simulink model "acc_RR_backup"  (R2021b)
settings: Solver=FixedStepAuto  StartTime=0.0  StopTime=40  FixedStep=0.0005  RelTol=1e-3
values from neighbouring files (symbols this model uses):
  s_path = [0 1.10508939428 2.2141958029 3.32141571172 4.42705301151 5.53154548532 6.63517443471 7.73808041313 8.84055018688 9.94289959674 11.0453539299 12.1480581097 ... (1001 elements, 1001x1)]    [200_100radius.mat]    (also in LV_Clothoid_S_Turn_path.mat = [0 0.966832089581 1.93621320584 2.90214024471 3.86476766313 ; NEDC_path.mat = [0 0.414605943146 0.832514087334 1.25401518562 1.68216660344; Straight_East_into_curve.mat = [0 1.65770560069 3.32192925577 4.98420060507 6.64484613518 8; acc_plot_backup.m = Station_HV_m)
  X_path = [0 1.10508939428 2.2141958029 3.32141571172 4.42705301151 5.53154548532 6.63517443471 7.73808041313 8.84055018688 9.94289959674 11.0453539299 12.1480581097 ... (1001 elements, 1001x1)]    [200_100radius.mat]    (also in LV_Clothoid_S_Turn_path.mat = [-10 -9.03316791042 -8.06378679416 -7.09785975529 -6.1352323; NEDC_path.mat = [0 0.414605943146 0.832514087334 1.25401518562 1.68216660344; Straight_East_into_curve.mat = [0 1.65770560069 3.32192925577 4.98420060507 6.64484613518 8; acc_plot_backup.m = X_HV_m)
  Y_path = [0 -1.70364610795e-18 -7.41532896709e-18 1.46822109542e-17 4.74557362791e-17 6.12980216762e-17 9.25043977736e-17 1.24088240159e-16 1.5099156923e-16 1.7058517853e-16 1.90629227614e-16 2.09673434424e-16 ... (1001 elements, 1001x1)]    [200_100radius.mat]    (also in LV_Clothoid_S_Turn_path.mat = [0 -8.46153035536e-19 5.07382551045e-18 2.07356032218e-17 3.; NEDC_path.mat = [0 -3.50680326162e-18 -2.14111304971e-18 3.38197671014e-18 3; Straight_East_into_curve.mat = [0 1.29197709199e-18 2.81882429322e-18 3.49020462564e-17 6.7; acc_plot_backup.m = Y_HV_m)
undefined symbols (not defined in the file or in its folder): C_TICK_TIME_S, ENUM_ACCSTATE_DISABLED, ENUM_ACCSTATE_OFF, ENUM_ACCSTATE_STANDBY, FALSE, KVDI_ACCLongPressTime_ms, KVDI_ACCMaxActSpeed_kph, KVDI_ACCSetSpdIntial_kph, KVDI_ACCSpdLargeChange_kph, KVDI_LongPressConTime_ms, ONE_FLOAT, ONE_INT, R, Rw, T, TRUE, ZERO_FLOAT, ZERO_INT
libraries: simulink x15, simulink_extras x2, Solver_SF x1
(part 1 of 4)
settings Model: Creator=power  LastModifiedBy=power
settings DataIOCC: ReturnWorkspaceOutputs=off

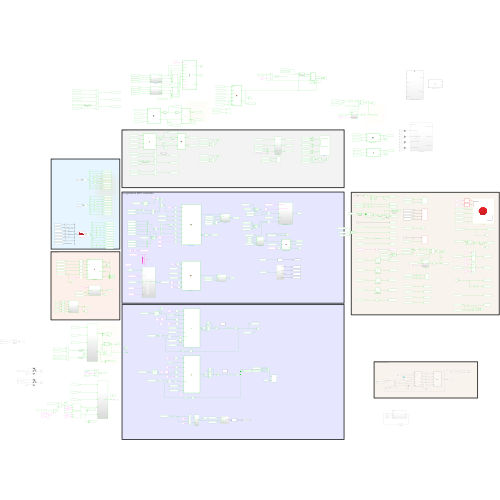
[thumbnail: Simulink's stored preview of the top-level diagram]
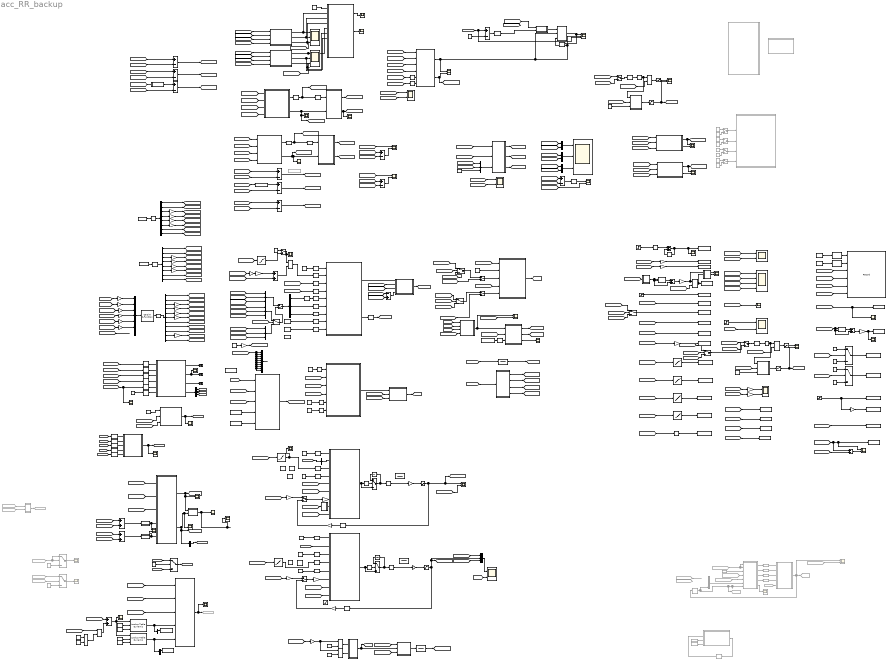
== system acc_RR_backup ==
  note: Lateral MPC controller
  note: Kalman Filter
  note: Carsim
  note: Record data
  note: Longitudinal MPC controller
  note: Camera_emulator
  note: Longitudinal Constraint MPC controller
  1-D Lookup Table : Lookup_n-D  NumberOfTableDimensions=1  BreakpointsForDimension1=[-10:1]  Table=[2.4 2.4 2.3 2.2 2.1 2.0 1.9 1.8 1.7 1.6 1.5 1.5]  InternalRulePriority=Speed  RndMeth=Simplest  InputSameDT=on
  1-D Lookup Table Accel Limit1 : Lookup_n-D  NumberOfTableDimensions=1  BreakpointsForDimension1=[0,5,20,30]  Table=[4,4,2,2]  InternalRulePriority=Speed  RndMeth=Simplest  InputSameDT=on
  1-D Lookup Table Deccel Limit2 : Lookup_n-D  NumberOfTableDimensions=1  BreakpointsForDimension1=[0,5,20,30]  Table=[-5,-5,-2.5,-2.5]  InternalRulePriority=Speed  RndMeth=Simplest  InputSameDT=on
  1-D Lookup Table Jerk LowLimit1 : Lookup_n-D  NumberOfTableDimensions=1  BreakpointsForDimension1=[0,5,20,30]  Table=[-5,-5,-2.5,-2.5]  InternalRulePriority=Speed  RndMeth=Simplest  InputSameDT=on
  1-D Lookup Table Jerk UpLimit1 : Lookup_n-D  NumberOfTableDimensions=1  BreakpointsForDimension1=[0,5,20,30]  Table=[5,5,2.5,2.5]  InternalRulePriority=Speed  RndMeth=Simplest  InputSameDT=on
  1-D Lookup Table1 : Lookup_n-D  NumberOfTableDimensions=1  BreakpointsForDimension1=[35 40 70 80]/3.6  Table=[0.01 0.01 0.0025 0.0025]  InternalRulePriority=Speed  RndMeth=Simplest  InputSameDT=on
  1-D Lookup Table2 : Lookup_n-D  NumberOfTableDimensions=1  BreakpointsForDimension1=[0 10 35 40]/3.6  Table=[0.25 0.25 0.025 0.025]  InternalRulePriority=Speed  RndMeth=Simplest  InputSameDT=on
  ACCSpdCalculation : Subsystem  Commented=on
  ACC_Mode_Selector : Subsystem
  Abs{,1..3} (4 alike) : Abs
  Acceleration controller2 : MATLAB Function  TreatAsAtomicUnit=on
  Add{,1..3,5,13..18} (11 alike) : Sum  Inputs=+-
  Add Constant : Bias  Bias=-2
  Add Constant1 : Bias  Bias=2
  Add Constant2 : Bias  Bias=-2
  Add Constant3 : Bias  Bias=-4.5
  Add10 : Sum  Inputs=-+
  Add{6..9,11} (5 alike) : Sum
  Add12 : Sum  Inputs=-+
  Add4 : Sum  Inputs=-+
  Camera_NEW : MATLAB Function  TreatAsAtomicUnit=on
  CarSim S-Function : Solver_SF/CarSim S-Function  Priority=1  SIMFILE=simfile.sim  Run_RTs=off  vs_state_ind=Run  StopMode_ind=Vehicle Model
  Compare To Constant : simulink/Logic and Bit Operations/Compare To Constant  relop=<=  const=-0.2  OutDataTypeStr=boolean
  Constant{,8..9,16,19,28,40,42,52,58,92} (11 alike) : Constant
  Constant1 : Constant  Value=0
  Constant10 : Constant  Value=0.1
  Constant11 : Constant  Value=90
  Constant111 : Constant  Value=10
  Constant{12..13,24,45} (4 alike) : Constant  Commented=on  OutDataTypeStr=boolean
  Constant14 : Constant  Value=1270+22*4+88.6+54.4
  Constant{15,39,46..47} (4 alike) : Constant  Commented=on  Value=0  OutDataTypeStr=boolean
  Constant17 : Constant  Value=0.3
  Constant18 : Constant  Value=0.025
  Constant2 : Constant  Value=2
  Constant20 : Constant  Value=s_path
  Constant21 : Constant  Value=X_path
  Constant22 : Constant  Value=s_path
  Constant23 : Constant  Value=Y_path
  Constant25 : Constant  Commented=on  Value=0.3
  Constant26 : Constant  Value=X_path
  Constant27 : Constant  Value=Y_path
  Constant29 : Constant  Value=1.5
  Constant3 : Constant  Value=0.1
  Constant30 : Constant  Value=35
  Constant31 : Constant  Value=3
  Constant32 : Constant  Value=30
  Constant33 : Constant  Value=5
  Constant34 : Constant  Value=-3
  Constant35 : Constant  Value=-5
  Constant36 : Constant  Value=1.5
  Constant37 : Constant  Commented=on  Value=0.1
  Constant38 : Constant  Value=0.025
  Constant4 : Constant  Value=0.0025
  Constant41 : Constant  Value=0.01
  Constant43 : Constant  Value=0.0125
  Constant44 : Constant  Commented=on  Value=100
  Constant48 : Constant  Commented=on  Value=100
  Constant49 : Constant  Value=[1:10]'
  Constant5 : Constant  Value=0.2
  Constant50 : Constant  Commented=on  Value=3
  Constant51 : Constant  Value=0.1
  Constant53 : Constant  Value=1.5
  Constant6 : Constant  Value=2.5
  Constant7 : Constant  Value=0
  Delay{,3..4,7} (4 alike) : Delay  DelayLength=1  SampleTime=0.1
  Delay1 : Delay  DelayLength=1  InitialConditionSource=Input port  SampleTime=0.1
      settings: InputPortMap=u0,p4
  Delay2 : Delay  DelayLength=1  InitialConditionSource=Input port  SampleTime=0.1
      settings: InputPortMap=u0,p4
  Delay5 : Delay  Commented=on  DelayLength=1  SampleTime=0.1
  Delay6 : Delay  DelayLength=1  InitialConditionSource=Input port  SampleTime=0.1
      settings: InputPortMap=u0,p4
  Delay8 : Delay  Commented=on  DelayLength=1  SampleTime=0.1
  Demux : Demux  Outputs=11
  Demux1 : Demux  Outputs=8
  Demux14 : Demux
  Demux2 : Demux  Outputs=[10]
  Demux3 : Demux  Outputs=3
  Demux4 : Demux  Outputs=[1 9]
  Demux5 : Demux  Outputs=[1 9]
  Demux6 : Demux  Outputs=[8 10 12]
  Demux7 : Demux  Outputs=8
  Divide : Product  Inputs=*/
  Divide1 : Product  Inputs=*/
  Estimation_TTCx_PV : MATLAB Function  TreatAsAtomicUnit=on
  Estimation_TTCx_PV1 : MATLAB Function  TreatAsAtomicUnit=on
  Estimation_TTCy_PV : MATLAB Function  Commented=on  TreatAsAtomicUnit=on
  From Workspace : FromWorkspace  VariableName=LV
  From Workspace1 : FromWorkspace  VariableName=APV
  From149 : From  Commented=on  GotoTag=Ax_HV_mps2
  From157 : From  Commented=on  GotoTag=Vx_p
  From159 : From  Commented=on  GotoTag=ACCSetSpeed_mps
  From160 : From  Commented=on  GotoTag=Vx_HV_mps
  From161 : From  Commented=on  GotoTag=Ax_HV_mps2
  From163 : From  Commented=on  GotoTag=RR
  From165 : From  Commented=on  GotoTag=xref
  From166 : From  Commented=on  GotoTag=yref
  From167 : From  Commented=on  GotoTag=xref
  From169 : From  Commented=on  GotoTag=xref
  From170 : From  Commented=on  GotoTag=yref
  From245 : From  Commented=on  GotoTag=ax_c_old
  Gain{1..2,5,9..10,15..16} (7 alike) : Gain  Gain=1/3.6
  Gain{3..4,6..7,11,29} (6 alike) : Gain  Gain=9.81
  Gain12 : Gain  Gain=0.5
  Gain{8,13,19..21,31} (6 alike) : Gain  Gain=3.6
  Gain14 : Gain  Gain=pi/180
  Gain17 : Gain  Gain=0.1
  Gain18 : Gain  Gain=[0:9]
  Gain22 : Gain  Gain=0.5
  Gain23 : Gain  Gain=20
  Gain{24..26,34} (4 alike) : Gain  Gain=1/20
  Gain27 : Gain  Gain=pi/180
  Gain28 : Gain  Gain=20
  Gain30 : Gain  Gain=pi/180
  Gain{33,36..38} (4 alike) : Gain
  Gain35 : Gain  Gain=-1
  Goto31 : Goto  Commented=on  GotoTag=ax_c_old
  Goto44 : Goto  Commented=on  GotoTag=spd_acc
  Goto46 : Goto  Commented=on  GotoTag=LeftDis_Camera
  Goto49 : Goto  Commented=on  GotoTag=LeftDis_PV
  Latch : Subsystem
  Logical Operator : Logic  Operator=NOT  AllPortsSameDT=off  OutDataTypeStr=boolean
  Lookup Table Dynamic : simulink/Lookup Tables/Lookup Table Dynamic  LookUpMeth=Interpolation-Use End Values  OutDataType=fixdt('double')  OutScaling=[]  OutputDataTypeScalingMode=Specify via dialog  OutDataTypeStr=double  DoSatur=off
  Lookup Table Dynamic1 : simulink/Lookup Tables/Lookup Table Dynamic  LookUpMeth=Interpolation-Use End Values  OutDataType=fixdt('double')  OutScaling=[]  OutputDataTypeScalingMode=Specify via dialog  OutDataTypeStr=double  DoSatur=off
  MATLAB Function : MATLAB Function  TreatAsAtomicUnit=on
  MATLAB Function1 : MATLAB Function  TreatAsAtomicUnit=on
  MATLAB Function10 : MATLAB Function  TreatAsAtomicUnit=on
  MATLAB Function13 : MATLAB Function  TreatAsAtomicUnit=on
  MATLAB Function17 : MATLAB Function  TreatAsAtomicUnit=on
  MATLAB Function2 : MATLAB Function  TreatAsAtomicUnit=on
  MATLAB Function3 : MATLAB Function  TreatAsAtomicUnit=on
  MATLAB Function4 : MATLAB Function  TreatAsAtomicUnit=on
  MATLAB Function5 : MATLAB Function  TreatAsAtomicUnit=on
  MATLAB Function6 : MATLAB Function  TreatAsAtomicUnit=on
  MATLAB Function7 : MATLAB Function  TreatAsAtomicUnit=on
  MATLAB Function8 : MATLAB Function  TreatAsAtomicUnit=on
  MPC : MATLAB Function  Commented=on  TreatAsAtomicUnit=on
  MPC_ACC : MATLAB Function  TreatAsAtomicUnit=on
  MPC_Bicycle_LDC1 : MATLAB Function  TreatAsAtomicUnit=on
  Manual Switch : ManualSwitch  Commented=on
  Manual Switch1 : ManualSwitch  CurrentSetting=0
  Manual Switch10 : ManualSwitch  Commented=on  CurrentSetting=0
  Manual Switch11 : ManualSwitch  Commented=on
  Manual Switch12 : ManualSwitch  Commented=on
  Manual Switch{2..6,8..9} (7 alike) : ManualSwitch
  Mux : Mux  Inputs=7
  Mux1 : Mux  Inputs=2
  Mux{4,6..8,10} (5 alike) : Mux  Inputs=3
  Mux2 : Mux  Inputs=2
  Mux3 : Mux  Inputs=2
  Mux5 : Mux  Inputs=10
  Mux9 : Mux  Commented=on  Inputs=[3 1 1 1]
  Product : Product
  Product1 : Product
  Product10 : Product
  QP_logitudinal1 : MATLAB Function  Commented=on  TreatAsAtomicUnit=on
  R1 : Constant  Value=0.5
  Radians to Degrees1 : simulink_extras/Transformations/Radians to Degrees
  Radians to Degrees2 : simulink_extras/Transformations/Radians to Degrees
  Rate Transition{1..5,18} (6 alike) : RateTransition  OutPortSampleTime=0.1
  Relational Operator : RelationalOperator  OutDataTypeStr=boolean  RndMeth=Simplest
  Relational Operator1 : RelationalOperator  Operator=<=  OutDataTypeStr=boolean  RndMeth=Simplest
  Relational Operator2 : RelationalOperator  Operator=isNaN  OutDataTypeStr=boolean  RndMeth=Simplest
  Relational Operator4 : RelationalOperator  Operator=isNaN  OutDataTypeStr=boolean  RndMeth=Simplest
  Saturation{,1,5..6} (4 alike) : Saturate  UpperLimit=2.5  LowerLimit=0
  Saturation2 : Saturate  UpperLimit=30/3.6  LowerLimit=5/3.6
  Saturation3 : Saturate  UpperLimit=720  LowerLimit=-720
  Saturation4 : Saturate  UpperLimit=400  LowerLimit=-400
  Scope{,1..2,5,8,13,17..20,25,27..28,30,42..44,46,67} (19 alike) : Scope  NumInputPorts=2
  Scope{3..4,6..7,9..10,14..16,22..24,26,29,31..32,35,37,39,41,45,159} (22 alike) : Scope
  Scope{11,36,40,47} (4 alike) : Scope  NumInputPorts=3
  Scope12 : Scope  NumInputPorts=4
  Scope21 : Scope  Commented=on  NumInputPorts=2
  Scope33 : Scope  Commented=on
  Scope34 : Scope  Commented=on
  Scope38 : Scope  Commented=on
  Smooth Switch : Subsystem
  Smooth Switch1 : Subsystem
  Step : Step  Time=0  Before=1.5  After=1.5  SampleTime=0
  Step1 : Step  Time=0  Before=1.5  After=1.5  SampleTime=0
  Step2 : Step  Time=0  After=0.1  SampleTime=0
  Step3 : Step  Time=0  Before=5  After=5  SampleTime=0.1
  Subsystem : Subsystem
  Subsystem1 : Subsystem
  Subsystem16 : Subsystem
  Subsystem17 : Subsystem
  Subsystem2 : Subsystem
  Subsystem20 : Subsystem
  Subsystem3 : Subsystem
  Subsystem4 : Subsystem
  Subsystem5 : Subsystem
  Subsystem6 : Subsystem  Commented=on
  Subsystem7 : Subsystem
  Subsystem8 : Subsystem
  Switch : Switch  Criteria=u2 > Threshold
  Switch{1,7..11} (6 alike) : Switch  Criteria=u2 ~= 0
  Switch2 : Switch  Commented=on  Criteria=u2 > Threshold
  Switch3 : Switch  Commented=on  Criteria=u2 > Threshold
  Switch4 : Switch  Criteria=u2 > Threshold
  Switch5 : Switch  Threshold=8
  Switch6 : Switch  Threshold=8
  TH_ref : Constant  Value=1.5
  Terminator1 : Terminator
  Terminator2 : Terminator
  Terminator3 : Terminator
  To Workspace : ToWorkspace  VariableName=X_HV_m  SampleTime=-1
  To Workspace1 : ToWorkspace  VariableName=Y_HV_m  SampleTime=-1
  To Workspace10 : ToWorkspace  VariableName=TH  SampleTime=-1
  To Workspace11 : ToWorkspace  VariableName=RR  SampleTime=-1
  To Workspace12 : ToWorkspace  VariableName=Desired_distance  SampleTime=-1
  To Workspace13 : ToWorkspace  VariableName=C_tick_time  SampleTime=-1
  To Workspace14 : ToWorkspace  VariableName=Ax_HV_mps2  SampleTime=-1
  To Workspace15 : ToWorkspace  VariableName=V_ref_kph  SampleTime=-1
  To Workspace16 : ToWorkspace  VariableName=Ax_Up_Limit  SampleTime=-1
  To Workspace17 : ToWorkspace  VariableName=Ax_Low_Limit  SampleTime=-1
  To Workspace18 : ToWorkspace  VariableName=Jerk_x_Up_Limit  SampleTime=-1
  To Workspace19 : ToWorkspace  VariableName=Jerk_x_Low_Limit  SampleTime=-1
  To Workspace2 : ToWorkspace  VariableName=Yaw_HV_deg  SampleTime=-1
  To Workspace20 : ToWorkspace  VariableName=Acc_Mode  SampleTime=-1
  To Workspace21 : ToWorkspace  VariableName=Ay_Low_Limit  SampleTime=-1
  To Workspace22 : ToWorkspace  VariableName=Jerk_y_Up_Limit  SampleTime=-1
  To Workspace23 : ToWorkspace  VariableName=Jerk_y_Low_Limit  SampleTime=-1
  To Workspace24 : ToWorkspace  VariableName=Ay_HV_mps2  SampleTime=-1
  To Workspace25 : ToWorkspace  VariableName=y_error  SampleTime=-1
  To Workspace26 : ToWorkspace  VariableName=Steer_SW_deg  SampleTime=-1
  To Workspace27 : ToWorkspace  VariableName=X_ref  SampleTime=-1
  To Workspace28 : ToWorkspace  VariableName=Y_ref  SampleTime=-1
  To Workspace3 : ToWorkspace  VariableName=Station_HV_m  SampleTime=-1
  To Workspace4 : ToWorkspace  VariableName=Jerk_y  SampleTime=-1
  To Workspace5 : ToWorkspace  VariableName=Ay_Up_Limit  SampleTime=-1
  To Workspace6 : ToWorkspace  VariableName=HV_kph  SampleTime=-1
  To Workspace7 : ToWorkspace  VariableName=PV_kph  SampleTime=-1
  To Workspace8 : ToWorkspace  VariableName=Jerk_x  SampleTime=-1
  To Workspace9 : ToWorkspace  VariableName=TH_ref  SampleTime=0.1
  Transfer Fcn{1..4} (4 alike) : TransferFcn  Denominator=[0.3 1]
  Unit Delay : UnitDelay  SampleTime=-1  HasFrameUpgradeWarning=on
  Unit Delay2 : UnitDelay  SampleTime=-1  HasFrameUpgradeWarning=on
  V_rel Estimation : Subsystem
  XY Graph : Record  FileSettingsInternal="{\"entries\":[{\"content\":{\"excelSettings\":{\"content\":{},\"type\":\"Streamout.ExcelSettings\"}},\"type\":\"Streamout.FileSettingStorage\",\"uuid\":\"a3c8dcb7-cd04-47db-8df7-74fc07aaeb0b\"}],\"packageUris\":[\"http://schema.mathworks.com/mf0/streamout_blocks/R2020a\"],\"version\":\"1.0\"}"  Layout=[1 1]  SignalsInternal="{\"entries\":[{\"content\":{\"signals\":[{\"content\":{\"blockPath\":[\"acc/XY Graph\"],\"channel\":[],\"dimensions\":[1],\"domain\":\"acc/XY Graph\",\"lineColor\":\"#a2142f\",\"plots\":[1],\"port\":1,\"sid\":[\"\"],\"signalID\":328902,\"signalName\":\"x\"},\"type\":\"RecordBlkView.Signal\",\"uuid\":\"58a908f8-b328-4002-bf13-044fef450135\"},{\"content\":{\"blockPath\":[\"acc/XY Graph\"],\"channel\":[],\"dimensions\":[1],\"domain\":\"acc/XY Graph\",\"lineColor\":\"#139fff\",\"plots\":[1],\"port\":2,\"sid\":[\"\"],\"signalID\":328906,\"signalName\":\"y\"},\"type\":\"RecordBlkView.Signal\",\"uuid\":\"8476c32c-9a1a-438a-a83a-d74f9b55deb6\"},{\"content\":{\"blockPath\":[\"acc/XY Graph\"],\"channel\":[],\"dimensions\":[1],\"domain\":\"acc/XY Graph\",\"lineColor\":\"#64d413\",\"plots\":[1],\"port\":3,\"sid\":[\"\"],\"signalID\":328910,\"signalName\":\"X_HV\"},\"type\":\"RecordBlkView.Signal\",\"uuid\":\"60bc389a-c242-4b2e-b286-84b9602f93c9\"},{\"content\":{\"blockPath\":[\"acc/XY Graph\"],\"channel\":[],\"dimensions\":[1],\"domain\":\"acc/XY Graph\",\"lineColor\":\"#ff13a6\",\"plots\":[1],\"port\":4,\"sid\":[\"\"],\"signalID\":328914,\"signalName\":\"Y_HV\"},\"type\":\"RecordBlkView.Signal\",\"uuid\":\"a6cb8bdb-3617-4429-b963-4035cabf589a\"},{\"content\":{\"blockPath\":[\"acc/XY Graph\"],\"channel\":[],\"dimensions\":[1],\"domain\":\"acc/XY Graph\",\"lineColor\":\"#ff6929\",\"plots\":[1],\"port\":5,\"sid\":[\"\"],\"signalID\":328918,\"signalName\":\"X_PV\"},\"type\":\"RecordBlkView.Signal\",\"uuid\":\"139bb408-47f9-477b-b130-41a093de5c1a\"},{\"content\":{\"blockPath\":[\"acc/XY Graph\"],\"channel\":[],\"dimensions\":[1],\"domain\":\"acc/XY Graph\",\"lineColor\":\"#b746ff\",\"plots\":[1],\"port\":6,\"sid\":[\"\"],\"signalID\":328922,\"signalName\":\"Y_PV\"},\"type\":\"RecordBlkView.Signal\",\"uuid\":\"dcabd0e2-8491-473f-998f-2ebadf0b1da2\"}]},\"type\":\"RecordBlkView.InputSignals\",\"uuid\":\"b146c4fa-b7cd-488d-8ce9-66e4c4b64d1a\"}],\"packageUris\":[\"http://schema.mathworks.com/mf0/streamout_blocks/R2020a\"],\"version\":\"1.0\"}"  VisualizationBindings="{\"xyplotplugin\":{\"info\":[{\"series\":[{\"bindingParametersList\":[{\"parameter\":\"X-Axis\",\"signalID\":328902,\"signalName\":\"x\"},{\"parameter\":\"Y-Axis\",\"signalID\":328906,\"signalName\":\"y\"}],\"seriesID\":43394},{\"bindingParametersList\":[{\"parameter\":\"X-Axis\",\"signalID\":328918,\"signalName\":\"X_PV\"},{\"parameter\":\"Y-Axis\",\"signalID\":328922,\"signalName\":\"Y_PV\"}],\"seriesID\":18431},{\"bindingParametersList\":[{\"parameter\":\"X-Axis\",\"signalID\":328910,\"signalName\":\"X_HV\"},{\"parameter\":\"Y-Axis\",\"signalID\":328914,\"signalName\":\"Y_HV\"}],\"seriesID\":48931}],\"subplotID\":1}]}}"  CompatibilityTag=XY
  Zero-Order Hold{1..14,17..25,132..136} (28 alike) : ZeroOrderHold  SampleTime=0.1
  Zero-Order Hold{26..27,29,36} (4 alike) : ZeroOrderHold  Commented=on  SampleTime=0.1
  acceleration_apr1 : Subsystem
  acceleration_apr4 : Subsystem
  car_length : Bias  Bias=-4.5
  car_length1 : Bias  Bias=4.5
  car_length2 : Bias  Bias=-4.5
  car_length3 : Bias  Bias=4.5
  cmd_limiter2 : Subsystem
  cmd_limiter3 : Subsystem
  demux : Subsystem
  demux2 : Subsystem
  dist_safe : Bias  Bias=-2
  divide : Subsystem
  divide1 : Subsystem
  global to local1 : Subsystem
  global to local3 : Subsystem
  relative_dynamic_estimated : Subsystem  Commented=on
  rolling_avg : Subsystem  Commented=on
  sample time1 : Gain  Gain=1/0.1
  sample time2 : Gain  Gain=1/0.1
  velocity_apr5 : Subsystem  Commented=on
  wires:
  V_rel Estimation/3(a_rel) -> [a_Rel_est]
  [RR] -> V_rel Estimation/2(S_rel)
  [Ax_HV_mps2] -> V_rel Estimation/1(a_c)
  V_rel Estimation/1(s_rel) -> [S_Rel_est]
  Demux/1 -> [X_HV_m]
  CarSim S-Function/1 -> Zero-Order Hold18/1
  Demux/2 -> [Y_HV_m]
  Demux/3 -> Gain9/1
  Demux/4 -> Gain10/1
  Demux/5 -> Gain3/1
  Demux/6 -> Gain4/1
  From Workspace/1 -> Zero-Order Hold5/1
  Demux1/1 -> [X_PV_m]
  Demux1/6 -> Gain11/1
  Demux1/5 -> Gain7/1
  Demux1/4 -> Gain2/1
  Demux1/3 -> Gain1/1
  Demux1/2 -> [Y_PV_m]
  Divide/1 -> Saturation/1  "TH_cal"
  Saturation/1 -> Scope5/1  "TH"
  [Vx_PV_mps] -> Add1/1
  [Vx_HV_mps] -> Add1/2
  acceleration_apr4/1(acc_a) -> Add2/1  "PV"
  [Ax_HV_mps2] -> Add2/2  "HV"
  Constant14/1 -> Zero-Order Hold17/1
  Subsystem2/4(Pb_RR) -> [Braking_Pressure_RR]
  Product/1 -> Zero-Order Hold6/1
  [Driving_Brk_Cmd] -> Subsystem2/1(T_cmd)
  Subsystem2/1(Pb_LF) -> [Braking_Pressure_LF]
  Acceleration controller2/2(Tb) -> [Driving_Brk_Cmd]
  Acceleration controller2/3(Rtotal) -> Scope159/1
  Subsystem2/3(Pb_RL) -> [Braking_Pressure_RL]
  [Ax_HV_mps2] -> Zero-Order Hold9/1
  [Vx_HV_mps] -> Zero-Order Hold8/1
  Acceleration controller2/1(Tr) -> [Driving_Torque_Cmd]  "Torque"
  Subsystem2/2(Pb_RF) -> [Braking_Pressure_RF]
  Gain9/1 -> [Vx_HV_mps]
  Gain10/1 -> [Vy_HV_mps]
  Gain2/1 -> [Vy_PV_mps]
  Gain3/1 -> [Ax_HV_mps2]
  Gain4/1 -> [Ay_HV_mps2]
  Gain11/1 -> [Ay_PV_mps2]
  Gain22/1 -> Mux/1  "Driving_Torque_FL"
  Gain12/1 -> Mux/2  "Driving_Torque_FR"
  Zero-Order Hold6/1 -> MATLAB Function1/2(Yref)
  Zero-Order Hold8/1 -> MATLAB Function1/3(Vx)
  Zero-Order Hold9/1 -> MATLAB Function1/4(ax)
  Zero-Order Hold10/1 -> MATLAB Function1/5(D_rel)
  Zero-Order Hold11/1 -> MATLAB Function1/6(V_rel)
  Zero-Order Hold12/1 -> MATLAB Function1/7(ax_rel)
  Zero-Order Hold13/1 -> MATLAB Function1/8(Qs)
  Zero-Order Hold14/1 -> MATLAB Function1/9(Rs)
  Abs/1 -> divide/1(dividend), Divide/1
  Mux1/1 -> Scope11/1  "RR"
  [RR] -> Mux1/1  "RR"
  [S_Rel_est] -> Mux1/2  "Est"
  [RVx] -> Mux2/1  "RV"
  [V_Rel_est] -> Mux2/2  "Est"
  [RAx] -> Mux3/1  "RA"
  [a_Rel_est] -> Mux3/2  "Est"
  Mux2/1 -> Scope11/2  "RV"
  Mux3/1 -> Scope11/3  "RA"
  [Braking_Pressure_RF] -> Gain36/1
  Gain33/1 -> Mux/3  "Driving_Torque_LF"
  [Braking_Pressure_LF] -> Gain33/1
  [Braking_Pressure_RL] -> Gain37/1
  Gain36/1 -> Mux/4  "Driving_Torque_RF"
  Gain38/1 -> Mux/6  "Driving_Torque_RR"
  Gain37/1 -> Mux/5  "Driving_Torque_RL"
  [Braking_Pressure_RR] -> Gain38/1
  [Braking_Pressure_LF] -> Scope12/1  "LF"
  [Braking_Pressure_RF] -> Scope12/2  "RF"
  [Braking_Pressure_RL] -> Scope12/3  "RL"
  [Braking_Pressure_RR] -> Scope12/4  "RR"
  MATLAB Function1/2(Y) -> Add Constant1/1  "MPC"
  Gain8/1 -> Scope18/1  "HV"
  Gain13/1 -> Scope18/2  "PV"
  Zero-Order Hold5/1 -> Demux1/1
  [Vx_HV_mps] -> Acceleration controller2/2(Vxh)
  Zero-Order Hold17/1 -> Acceleration controller2/3(m)
  Zero-Order Hold18/1 -> Demux/1
  [RR] -> Scope13/2  "RR"
  [Vx_HV_mps] -> Divide/2
  Mux4/1 -> V_rel Estimation/3(initial_value)
  [RR] -> Mux4/1
  Constant7/1 -> Mux4/3
  Step/1 -> Scope2/1  "TH_limit"
  [TH] -> Scope2/2  "TH"
  Gain7/1 -> [Ax_PV_mps2]
  Demux3/3 -> Zero-Order Hold12/1
  Zero-Order Hold3/1 -> MATLAB Function1/1(mode)
  [Driving_Torque] -> Gain22/1
  [Driving_Torque] -> Gain12/1
  [Ax_HV_mps2] -> Scope17/2  "ax_out"
  [Vx_HV_mps] -> Gain8/1  "HV"
  [Vx_PV_mps] -> Gain13/1  "PV"
  Demux3/2 -> Zero-Order Hold11/1
  [Driving_Torque_Cmd] -> Transfer Fcn1/1
  Gain1/1 -> [Vx_PV_mps]
  [Vx_HV_mps] -> MPC_ACC/3(Vx)
  [Ax_HV_mps2] -> MPC_ACC/4(ax)
  Constant92/1 -> Zero-Order Hold1/1
  Constant5/1 -> Zero-Order Hold2/1
  Constant2/1 -> Subsystem/4(Ax_max)
  Constant6/1 -> Subsystem/5(Jx_max)
  [Vx_HV_mps] -> Subsystem/3(VehSpd)
  [Vx_p] -> MPC_ACC/2(vx_p)
  Subsystem/1("VREF_LongiVehSpdRef_mps ") -> [Vx_p]  "mps"
  Zero-Order Hold1/1 -> MPC_ACC/5(Qs)
  Zero-Order Hold2/1 -> MPC_ACC/6(Rs)
  V_rel Estimation/2(v_rel) -> [V_Rel_est]
  MATLAB Function1/1(u) -> cmd_limiter2/1(ax_cmd)  "cmd"
  [RVx] -> Mux4/2
  Constant28/1 -> Zero-Order Hold4/1
  Add2/1 -> [RAx]
  Add1/1 -> [RVx]
  [Acc_Mode] -> Subsystem/1("Trig ")
  [RR] -> ?
  [ACCSetSpeed_mps] -> Mux5/10, Mux5/9, Mux5/8, Mux5/7, Mux5/6, Mux5/5, Mux5/4, Mux5/3, Mux5/2, Mux5/1
  Add Constant/1 -> Abs/1
  Constant11/1 -> Gain15/1
  Gain15/1 -> [ACCSetSpeed_mps]
  Constant58/1 -> Zero-Order Hold3/1
  Demux3/1 -> dist_safe/1
  [ACCSetSpeed_mps] -> ACC_Mode_Selector/1(ACCSetSpeed_mps)
  Constant1/1 -> ACC_Mode_Selector/2(VACCTargetVehNotAssigned_flg)
  [RR] -> Switch9/3
  [Vx_HV_mps] -> ACC_Mode_Selector/4(Vx_HV_mps)
  [RVx] -> Switch8/3
  [Vx_HV_mps] -> Add6/2
  [Ax_HV_mps2] -> Gain17/1
  Gain17/1 -> Gain18/1
  Gain18/1 -> Add6/1
  Add6/1 -> Product/2  "Vp"
  Add Constant1/1 -> [Desired_distance]
  [Ax_PV_mps2] -> acceleration_apr4/1(acc_b)  "PV"
  Transfer Fcn1/1 -> [Driving_Torque]
  [Vx_PV_mps] -> Gain19/1  "PV"
  [Vx_HV_mps] -> Gain20/1  "HV"
  Gain19/1 -> To Workspace7/1  "PV"
  Gain20/1 -> To Workspace6/1  "HV"
  Subsystem4/1(new_ave) -> Delay2/1, Delay2/2, Add10/2
  Add10/1 -> sample time1/1
  Delay2/1 -> Add10/1
  sample time1/1 -> Scope28/1, Subsystem3/1(Jerk)  "Jerk"
  Step1/1 -> To Workspace9/1  "TH_limit"
  [TH] -> To Workspace10/1  "TH"
  Switch10/1 -> To Workspace11/1  "RR"
  [Desired_distance] -> Scope13/1  "Desired_distance"
  [Desired_distance] -> To Workspace12/1  "Desired_distance"
  Step2/1 -> Delay3/1
  Add11/1 -> Scope31/1, To Workspace13/1, Delay/1
  Delay/1 -> Add11/2
  Delay3/1 -> Add11/1
  [Ax_HV_mps2] -> To Workspace14/1
  [ACCSetSpeed_mps] -> Subsystem/2(VehSpd_Ref)
  [ACCSetSpeed_mps] -> Gain21/1
  Gain21/1 -> To Workspace15/1
  Mux5/1 -> ?
  Constant30/1 -> Relational Operator/2
  Relational Operator1/1 -> Latch/2(reset)
  Constant32/1 -> Relational Operator1/2
  Relational Operator/1 -> Latch/1(set)
  Gain31/1 -> Relational Operator/1, Relational Operator1/1  "kph"
  [RR] -> Estimation_TTCx_PV/1(R)
  [RVx] -> Estimation_TTCx_PV/2(V)
  [RAx] -> Estimation_TTCx_PV/3(A)
  Estimation_TTCx_PV/1(TTC1) -> Scope27/1, [TTC_PV]
  Estimation_TTCx_PV/2(TTC2) -> Scope27/2
  [Vx_HV_mps] -> 1-D Lookup Table Deccel Limit2/1
  1-D Lookup Table Deccel Limit2/1 -> To Workspace17/1
  [Vx_HV_mps] -> 1-D Lookup Table Accel Limit1/1
  1-D Lookup Table Accel Limit1/1 -> To Workspace16/1
  [Vx_HV_mps] -> 1-D Lookup Table Jerk UpLimit1/1
  [Vx_HV_mps] -> 1-D Lookup Table Jerk LowLimit1/1
  1-D Lookup Table Jerk UpLimit1/1 -> To Workspace18/1
  1-D Lookup Table Jerk LowLimit1/1 -> To Workspace19/1
  dist_safe/1 -> Zero-Order Hold10/1  "Drel"
  [Acc_Mode] -> Logical Operator/1
  Constant29/1 -> divide/3(default_value)
  divide/1(quotient) -> Saturation1/1
  Saturation1/1 -> [TH], Scope5/2  "TH_default"
  [X_PV_m] -> MATLAB Function3/1(Xf)
  [Y_PV_m] -> MATLAB Function3/2(Yf)
  [X_HV_m] -> MATLAB Function3/3(Xh)
  [Y_HV_m] -> MATLAB Function3/4(Yh)
  MATLAB Function3/1(RR) -> car_length/1  "RR_XY"
  Demux/7 -> [Station_HV_m]  "Station_HV"
  Demux1/7 -> [Station_PV_m]
  [Station_HV_m] -> Add15/2
  [Station_PV_m] -> Add15/1
  Add15/1 -> Add Constant3/1  "station"
  Add Constant3/1 -> Scope67/1
  Constant9/1 -> Zero-Order Hold13/1
  Constant10/1 -> Zero-Order Hold14/1
  [a_Rel_est] -> Mux6/3
  [V_Rel_est] -> Mux6/2
  [S_Rel_est] -> Mux6/1
  [RR] -> Mux7/1
  [RVx] -> Mux7/2
  [RAx] -> Mux7/3
  Manual Switch1/1 -> Demux3/1
  Mux6/1 -> Manual Switch1/1
  Mux7/1 -> Switch7/3
  [S_Rel_est] -> Manual Switch3/2
  Manual Switch3/1 -> Add Constant/1
  Zero-Order Hold4/1 -> MPC_ACC/1(trig)
  [S_Rel_est] -> Manual Switch2/2
  Manual Switch2/1 -> ACC_Mode_Selector/3(RR)
  [Acc_Mode] -> Scope6/1
  Smooth Switch/1(ax_cmd) -> Acceleration controller2/1(axc), Scope17/1
  Manual Switch4/1 -> ACC_Mode_Selector/5(RV)
  [V_Rel_est] -> Manual Switch4/2
  [Vx_HV_mps] -> divide/2(divisor)
  [Ax_HV_mps2] -> Scope20/2  "HV"
  [Ax_PV_mps2] -> Scope20/1  "PV"
  car_length/1 -> [RR], car_length1/1  "RR"
  [RR] -> Scope67/2
  Demux/8 -> [Steer_SW_deg]
  Rate Transition1/1 -> Camera_NEW/4(Yo)
  Demux14/3 -> [C2]
  Rate Transition3/1 -> Camera_NEW/2(phi_deg)
  [PrediDis] -> Zero-Order Hold136/1
  [Y_HV_m] -> Rate Transition1/1
  [X_HV_m] -> Rate Transition2/1
  [Yaw_HV_deg] -> Rate Transition3/1  "deg"
  [Station_HV_m] -> Scope14/1, Rate Transition18/1
  Rate Transition2/1 -> Camera_NEW/3(Xo)
  Rate Transition18/1 -> Camera_NEW/5(station)
  Zero-Order Hold134/1 -> Subsystem16/3("C2 ")
  [C2] -> Zero-Order Hold134/1
  [C3] -> Zero-Order Hold135/1
  Camera_NEW/3(Heading_ref) -> Terminator2/1
  [C0] -> Zero-Order Hold132/1
  Rate Transition4/1 -> Camera_NEW/1(ux_mps)
  Demux14/1 -> [C0]
  Zero-Order Hold133/1 -> Subsystem16/2(C1)
  Zero-Order Hold135/1 -> Subsystem16/4(C3)
  Subsystem17/1(PrediDis) -> Scope15/1, [PrediDis]
  Zero-Order Hold136/1 -> Subsystem16/5(PrediDis)
  [Vx_HV_mps] -> Rate Transition4/1  "mps"
  Subsystem16/1(LeftDis) -> [LeftDis_Camera], Scope3/1
  [C1] -> Zero-Order Hold133/1
  Camera_NEW/1(x_ref) -> Terminator1/1
  Constant111/1 -> Subsystem17/1(Np)
  Camera_NEW/4(C) -> Demux14/1
  Demux14/2 -> [C1]
  Demux14/4 -> [C3]
  Zero-Order Hold132/1 -> Subsystem16/1(C0)
  Demux/9 -> [Yaw_HV_deg]
  [X_HV_m] -> To Workspace/1
  [Y_HV_m] -> To Workspace1/1
  [Yaw_HV_deg] -> To Workspace2/1
  [Station_HV_m] -> To Workspace3/1
  Rate Transition5/1 -> Camera_NEW/6(Ts_MPC)
  Constant3/1 -> Rate Transition5/1
  Zero-Order Hold19/1 -> MATLAB Function17/1(trig)
  Constant16/1 -> Zero-Order Hold19/1
  [y_ref] -> MATLAB Function17/2(Yref)
  Zero-Order Hold20/1 -> MATLAB Function17/3(tau)
  Constant17/1 -> Zero-Order Hold20/1
  Zero-Order Hold22/1 -> MATLAB Function17/5(Rs)
  Zero-Order Hold21/1 -> MATLAB Function17/4(Qs)
  Constant19/1 -> Zero-Order Hold22/1
  1-D Lookup Table2/1 -> Zero-Order Hold21/1
  Gain14/1 -> MATLAB Function17/6(steer_angle)
  Switch/1 -> Radians to Degrees1/1, Unit Delay/1
  Saturation3/1 -> Mux8/2, [Steer_Kinematic_deg], Delay4/1  "Kinematic"
  [Steer_SW_deg] -> Mux8/3  "carsim"
  Gain23/1 -> Saturation3/1  "deg"
  Delay4/1 -> Gain24/1
  Gain24/1 -> Manual Switch5/2  "deg"
  [Ax_HV_mps2] -> MATLAB Function17/8(Ax)
  Constant20/1 -> Lookup Table Dynamic/2
  Constant21/1 -> Lookup Table Dynamic/3
  Lookup Table Dynamic/1 -> Demux4/1, global to local3/4(X_ref)
  Add9/1 -> Lookup Table Dynamic1/1, Scope7/1, Lookup Table Dynamic/1
  Constant23/1 -> Lookup Table Dynamic1/3
  Constant22/1 -> Lookup Table Dynamic1/2
  Lookup Table Dynamic1/1 -> Demux5/1, global to local3/5(Y_ref)
  [X_HV_m] -> global to local3/1(Xc)
  [Yaw_HV_deg] -> global to local3/3(Yaw)  "deg"
  [Y_HV_m] -> global to local3/2(Yc)
  [Steer_IN_deg] -> ?
  MATLAB Function17/1(u) -> Relational Operator2/1, Switch/3
  Unit Delay/1 -> Switch/1
  Relational Operator2/1 -> Switch/2
  Demux/10 -> Gain30/1
  Gain30/1 -> [Yaw_rate_radps]
  Constant26/1 -> MATLAB Function13/1(u)
  MATLAB Function13/1(y) -> XY Graph/1  "x"
  Constant27/1 -> MATLAB Function5/1(u)
  MATLAB Function5/1(y) -> XY Graph/2  "y"
  [X_HV_m] -> XY Graph/3  "X_HV"
  [Y_HV_m] -> XY Graph/4  "Y_HV"
  [Vx_HV_mps] -> Gain31/1
  [Steer_SW_deg] -> Gain34/1  "carsim"
  Gain34/1 -> Manual Switch5/1  "deg"
  Manual Switch5/1 -> Gain14/1
  Latch/1(latched) -> Smooth Switch1/2(Mode), [LFC_Mode]
  [Ay_HV_mps2] -> To Workspace24/1, Scope9/1
  sample time2/1 -> To Workspace4/1, Scope10/1  "Jerk"
  Delay6/1 -> Add4/1
  Add4/1 -> sample time2/1
  [Ay_HV_mps2] -> Add4/2, Delay6/2, Delay6/1
  [Vx_HV_mps] -> Switch5/2
  Switch5/1 -> To Workspace5/1
  Constant31/1 -> Switch5/1
  Constant33/1 -> Switch5/3
  Constant35/1 -> Switch6/3
  Constant34/1 -> Switch6/1
  Switch6/1 -> To Workspace21/1
  [Vx_HV_mps] -> Switch6/2
  Step3/1 -> Gain35/1, To Workspace22/1  "TH_limit"
  Gain35/1 -> To Workspace23/1
  rolling_avg/1(new_ave) -> Delay5/1
  [Steer_SW_deg] -> To Workspace26/1  "carsim"
  1-D Lookup Table/1 -> Manual Switch8/2
  [V_Rel_est] -> 1-D Lookup Table/1
  Constant36/1 -> Manual Switch8/1
  Manual Switch8/1 -> Product/1, Scope4/1
  ACC_Mode_Selector/1(Out1) -> [Acc_Mode]
  [Y_HV_m] -> global to local1/2(Yc)
  [X_HV_m] -> global to local1/1(Xc)
  [Yaw_HV_deg] -> global to local1/3(Yaw)  "deg"
  Delay5/1 -> rolling_avg/2(old_ave)
  Constant37/1 -> rolling_avg/3(delta_t)  "T"
  Constant25/1 -> rolling_avg/4(tc)
  Smooth Switch1/1(ax_cmd) -> Transfer Fcn2/1
  Demux/11 -> [y_error_m]
  [y_error_m] -> Add/1, Scope19/1, To Workspace25/1  "HV"
  demux/1(X_ref) -> Scope30/2, global to local1/5(Y_ref)  "PV_9delay"
  demux2/1(X_ref) -> Scope30/1, global to local1/4(X_ref)
  Demux1/8 -> [y_error_LV]
  [y_error_LV] -> Add/2
  Add/1 -> Scope19/2  "add_PV"
  global to local1/1(x_ref) -> [xref], Scope22/1, MATLAB Function/1(x)
  global to local1/2(y_ref) -> Demux6/1, [yref], Scope32/1, MATLAB Function/2(y)
  Subsystem1/1(Out1) -> MPC_Bicycle_LDC1/8(Vx)
  Gain26/1 -> Manual Switch9/1  "deg"
  Manual Switch9/1 -> Gain27/1
  [Steer_SW_deg] -> Gain26/1  "carsim"
  Relational Operator4/1 -> Switch4/2
  Unit Delay2/1 -> Switch4/1
  MPC_Bicycle_LDC1/1(u) -> Switch4/3, Relational Operator4/1
  Gain25/1 -> Manual Switch9/2  "deg"
  Switch4/1 -> Unit Delay2/1, Radians to Degrees2/1
  Saturation4/1 -> [Steer_Dynamic_deg], Scope25/1, Delay7/1  "mpc"
  Delay7/1 -> Gain25/1
  [Ax_HV_mps2] -> MPC_Bicycle_LDC1/9(Ax)
  [Vx_HV_mps] -> Subsystem1/1(In1)
  Gain27/1 -> MPC_Bicycle_LDC1/7(steer_angel)
  Gain28/1 -> Saturation4/1  "deg"
  [Yaw_rate_radps] -> MPC_Bicycle_LDC1/6(yaw_rate)
  [Vy_HV_mps] -> MPC_Bicycle_LDC1/5(Vy)
  Zero-Order Hold24/1 -> MPC_Bicycle_LDC1/4(Rs)
  Zero-Order Hold23/1 -> MPC_Bicycle_LDC1/3(Qs)
  Constant42/1 -> Zero-Order Hold24/1
  1-D Lookup Table1/1 -> Scope16/1, Zero-Order Hold23/1
  [y_ref] -> Demux2/1
  Zero-Order Hold25/1 -> MPC_Bicycle_LDC1/1(trig)
  Constant40/1 -> Zero-Order Hold25/1
  [Steer_SW_deg] -> Scope25/2  "carsim"
  Constant46/1 -> Manual Switch12/1
  Constant45/1 -> Manual Switch12/2
  Manual Switch12/1 -> ACCSpdCalculation/5(VDINR_ACCSpdResInc_flg)
  Manual Switch11/1 -> ACCSpdCalculation/4(VDINR_ACCSpdSetDec_flg)
  Constant24/1 -> Manual Switch11/2
  Constant39/1 -> Manual Switch11/1
  Manual Switch10/1 -> ACCSpdCalculation/3(NVDI_ACCSystemStatePrev_enum)
  Constant15/1 -> Manual Switch10/1
  Constant13/1 -> Manual Switch10/2
  Manual Switch/1 -> ACCSpdCalculation/2(NVDI_ACCActingPrev_flg)
  Constant12/1 -> Manual Switch/2
  Constant47/1 -> Manual Switch/1
  Camera_NEW/2(y_ref) -> Scope26/1, Terminator3/1  "yref"
  MATLAB Function3/2(RD) -> [RD_PV], MATLAB Function10/2(RD), Scope35/1
  MATLAB Function10/1(RX) -> [RX]
  MATLAB Function10/2(RY) -> [RY]
  [RX] -> Scope/1  "RX"
  [X_PV_m] -> Add3/1
  [X_HV_m] -> Add3/2
  Add3/1 -> Scope/2
  Add5/1 -> Scope8/2
  [Y_HV_m] -> Add5/2
  [Y_PV_m] -> Add5/1
  [RY] -> Scope8/1  "RY"
  car_length1/1 -> MATLAB Function10/1(RR)  "RR"
  [RY] -> Add7/1
  [RX] -> Add8/1
  [X_HV_m] -> Add8/2
  [Y_HV_m] -> Add7/2
  Add7/1 -> demux/1(In1)  "Y_PV_m"
  Add8/1 -> demux2/1(In1)  "X_PV_m"
  Switch1/1 -> [y_ref]
  [LeftDis_Camera] -> Switch1/1
  [LeftDis_PV] -> Switch1/3
  Constant/1 -> Switch1/2  "LaneAvail_flg"
  [X_PV_m] -> XY Graph/5  "X_PV"
  [Y_PV_m] -> XY Graph/6  "Y_PV"
  [Steer_Dynamic_deg] -> Mux8/1  "Dynamic"
  Mux8/1 -> Scope1/1
  [Vx_HV_mps] -> Subsystem17/2(VehSpd_mps)
  Mux/1 -> CarSim S-Function/1
  cmd_limiter3/1(ax_cmd1) -> [spd_acc]
  cmd_limiter2/1(ax_cmd1) -> [th_acc]
  [Vx_HV_mps] -> cmd_limiter2/2(Vx_HV_mps)
  [TTC_PV] -> cmd_limiter2/3(TTC)
  From163/1 -> ?
  Zero-Order Hold27/1 -> QP_logitudinal1/3(A_cons)
  MPC/3(M_act) -> Zero-Order Hold27/1
  Delay8/1 -> Mux9/4, MPC/7(ax_c_old), Goto31/1
  Zero-Order Hold26/1 -> QP_logitudinal1/2(f)
  MPC/4(gamma_act) -> Zero-Order Hold29/1
  From160/1 -> MPC/4(vxh)
  MPC/1(HH) -> Zero-Order Hold36/1
  From159/1 -> MPC/1(vx_p), MPC/2(vx_acc_set)
  Zero-Order Hold29/1 -> QP_logitudinal1/4(b)
  MPC/5(fesible_flag) -> Scope38/1
  Mux9/1 -> MPC/6(X_thk)
  Constant50/1 -> MPC/3(mode)
  MPC/2(ff) -> Zero-Order Hold26/1
  From245/1 -> QP_logitudinal1/5(u_old)
  Zero-Order Hold36/1 -> QP_logitudinal1/1(H)
  QP_logitudinal1/1(u) -> Scope21/1, Goto44/1, Delay8/1
  From149/1 -> Scope21/2  "ax_out"
  From161/1 -> MPC/5(axh)
  [spd_acc] -> Smooth Switch/1(Spd_acc_cmd)  "cmd"
  [Acc_Mode] -> Smooth Switch/2(Mode)
  [th_acc] -> Smooth Switch/3(TH_acc_cmd)  "cmd"
  [TTC_PV] -> cmd_limiter3/3(TTC)
  [Vx_HV_mps] -> cmd_limiter3/2(Vx_HV_mps)
  MPC_ACC/1(u) -> cmd_limiter3/1(ax_cmd)  "cmd"
  [Steer_Dynamic_deg] -> Smooth Switch1/1(Dynamic_cmd)
  [Steer_Kinematic_deg] -> Smooth Switch1/3(Kinematic_cmd)
  [Vx_HV_mps] -> Subsystem3/2(Vx)
  Subsystem3/1(Out1) -> Subsystem5/1(new_value), To Workspace8/1
  [TTC_PV] -> Smooth Switch/4(TTC)
  [LFC_Mode] -> Scope1/2
  [Vx_HV_mps] -> 1-D Lookup Table1/1
  Radians to Degrees2/1 -> Gain28/1
  Radians to Degrees1/1 -> Gain23/1
  Demux2/1 -> MPC_Bicycle_LDC1/2(Yref)
  [Ax_HV_mps2] -> Subsystem17/3(In3)
  global to local3/1(y_path_ref10) -> Goto46/1, Scope24/1
  [Station_HV_m] -> Add9/1
  Constant51/1 -> Product1/2
  Product1/1 -> Product10/2
  Constant49/1 -> Product1/1
  Product10/1 -> Add9/2
  Demux4/1 -> To Workspace27/1
  Demux5/1 -> To Workspace28/1
  [Desired_distance] -> Add12/1
  [S_Rel_est] -> Add12/2
  Add12/1 -> cmd_limiter2/4(S_error)
  [Vx_HV_mps] -> 1-D Lookup Table2/1
  [Vx_HV_mps] -> MATLAB Function17/7(Vx)
  [Vx_HV_mps] -> Product10/1
  Transfer Fcn2/1 -> [Steer_IN_deg]
  Logical Operator/1 -> To Workspace20/1
  [Ax_HV_mps2] -> Subsystem4/1(new_value)
  Subsystem5/1(new_ave) -> Scope28/2
  MATLAB Function/1(yref) -> Scope29/1, Scope23/1
  Constant44/1 -> Switch2/3
  From165/1 -> Switch2/1, Switch2/2
  From167/1 -> Switch3/2
  Constant48/1 -> Switch3/3
  From166/1 -> Switch3/1
  Switch2/1 -> Scope33/1
  Switch3/1 -> Scope34/1
  Demux6/2 -> [LeftDis_PV]
  From170/1 -> Subsystem6/2(y)
  From169/1 -> Subsystem6/1(x)
  Subsystem6/1(Outport) -> Goto49/1
  [RR] -> Subsystem20/1(Rx)
  [RY] -> Subsystem20/2(Ry)
  [RVx] -> Subsystem20/3(RVx)
  [Vy_PV_mps] -> Add13/1
  [Vy_HV_mps] -> Add13/2
  Add13/1 -> [RVy]
  [RVy] -> Subsystem20/4(RVy)
  Subsystem20/1(theta_min) -> MATLAB Function2/2(theta_min_pv), Scope36/1
  Subsystem20/2(theta_max) -> MATLAB Function2/3(theta_max_pv), Scope36/2
  Subsystem20/3(Vectory_ang) -> MATLAB Function2/4(vector_pv)
  Constant52/1 -> MATLAB Function2/1(letgo_LC)
  MATLAB Function2/1(Vectory_pv) -> Scope37/1
  Demux7/8 -> [y_error_APV]
  Demux7/7 -> [Station_APV_m]
  Gain5/1 -> [Vx_APV_mps]
  Gain29/1 -> [Ax_APV_mps2]
  Zero-Order Hold7/1 -> Demux7/1
  Gain6/1 -> [Ay_APV_mps2]
  Gain16/1 -> [Vy_APV_mps]
  Demux7/2 -> [Y_APV_m]
  Demux7/3 -> Gain5/1
  Demux7/4 -> Gain16/1
  Demux7/5 -> Gain29/1
  Demux7/6 -> Gain6/1
  Demux7/1 -> [X_APV_m]
  From Workspace1/1 -> Zero-Order Hold7/1
  car_length3/1 -> MATLAB Function4/1(RR)  "RR"
  MATLAB Function4/2(RY) -> Scope45/1, [RY_APV]
  MATLAB Function4/1(RX) -> [RX_APV]
  car_length2/1 -> car_length3/1, [RR_APV]  "RR"
  MATLAB Function6/1(RR) -> car_length2/1  "RR_XY"
  [Y_HV_m] -> MATLAB Function6/4(Yh)
  [X_HV_m] -> MATLAB Function6/3(Xh)
  [Y_APV_m] -> MATLAB Function6/2(Yf)
  [X_APV_m] -> MATLAB Function6/1(Xf)
  Subsystem7/3(Vectory_ang) -> MATLAB Function2/7(vector_apv)
  Subsystem7/2(theta_max) -> MATLAB Function2/6(theta_max_apv), Scope40/2
  Subsystem7/1(theta_min) -> MATLAB Function2/5(theta_min_apv), Scope40/1
  [RVy_APV] -> Subsystem7/4(RVy)
  [RVx_APV] -> Subsystem7/3(RVx)
  [RY_APV] -> Subsystem7/2(Ry)
  [RR_APV] -> Subsystem7/1(Rx)
  MATLAB Function2/2(Vectory_apv) -> Scope41/1
  Add14/1 -> [RVx_APV]
  [Vx_HV_mps] -> Add14/2
  [Vx_APV_mps] -> Add14/1
  Add16/1 -> [RVy_APV]
  [Vy_HV_mps] -> Add16/2
  [Vy_APV_mps] -> Add16/1
  MATLAB Function6/2(RD) -> MATLAB Function4/2(RD), [RD_APV], Scope39/1
  [RR] -> Scope42/1  "RR"
  [RR_APV] -> Scope42/2  "RR_APV"
  [RD_APV] -> Scope40/3
  [RD_PV] -> Scope36/3
  Estimation_TTCx_PV1/2(TTC2) -> Scope43/2
  Estimation_TTCx_PV1/1(TTC1) -> [TTC_APV], Scope43/1
  [RAx_APV] -> Estimation_TTCx_PV1/3(A)
  [RVx_APV] -> Estimation_TTCx_PV1/2(V)
  [RR_APV] -> Estimation_TTCx_PV1/1(R)
  [Ax_APV_mps2] -> acceleration_apr1/1(acc_b)  "PV"
  Add17/1 -> [RAx_APV]
  [Ax_HV_mps2] -> Add17/2  "HV"
  acceleration_apr1/1(acc_a) -> Add17/1  "PV"
  Saturation5/1 -> Scope44/1  "TH"
  [Vx_HV_mps] -> divide1/2(divisor)
  divide1/1(quotient) -> Saturation6/1
  Add Constant2/1 -> Abs1/1
  [RR_APV] -> Manual Switch6/1
  Divide1/1 -> Saturation5/1  "TH_cal"
  Constant53/1 -> divide1/3(default_value)
  Manual Switch6/1 -> Add Constant2/1
  Saturation6/1 -> [TH_APV], Scope44/2  "TH_default"
  [S_Rel_est] -> Manual Switch6/2
  [Vx_HV_mps] -> Divide1/2
  Abs1/1 -> divide1/1(dividend), Divide1/1
  [RR] -> MATLAB Function7/1(RR_PV)  "RR"
  [RR_APV] -> MATLAB Function7/2(RR_APV)  "RR_APV"
  [RY_APV] -> MATLAB Function7/4(RY_APV)
  [RY] -> MATLAB Function7/3(RY_PV)
  [RD_PV] -> Abs2/1
  [RD_APV] -> Abs3/1
  MATLAB Function7/1(RR) -> Scope47/2, Delay1/2, MATLAB Function8/2(u), Scope46/1
  Abs2/1 -> MATLAB Function7/5(RD_PV)
  Abs3/1 -> MATLAB Function7/6(RD_APV)
  MATLAB Function7/2(trig) -> [cut_in_flg], Scope46/2
  [RAx_APV] -> Mux10/3
  [RVx_APV] -> Mux10/2
  [RR_APV] -> Mux10/1
  [cut_in_flg] -> Switch7/2
  Mux10/1 -> Switch7/1
  Switch7/1 -> Manual Switch1/2
  [cut_in_flg] -> Switch8/2
  [RVx_APV] -> Switch8/1
  Switch8/1 -> Manual Switch4/1
  [cut_in_flg] -> Switch9/2
  [RR_APV] -> Switch9/1
  Switch9/1 -> Manual Switch2/1
  [RR_APV] -> Switch10/1
  [cut_in_flg] -> Switch10/2
  [RR] -> Switch10/3  "RR"
  [RR] -> Switch11/3  "RR"
  [cut_in_flg] -> Switch11/2
  [RR_APV] -> Switch11/1
  Switch11/1 -> Manual Switch3/1  "RR"
  [TH] -> Scope47/3, Add18/1
  TH_ref/1 -> Add18/2
  Add18/1 -> Compare To Constant/1
  [TTC_APV] -> Subsystem8/1(TTC)
  Delay1/1 -> MATLAB Function8/3(old_u)
  Subsystem8/1(Out1) -> MATLAB Function8/1(tau)  "tau_selector"
  Compare To Constant/1 -> Subsystem8/2(Mode)
  MATLAB Function8/1(y) -> Delay1/1, Scope47/1

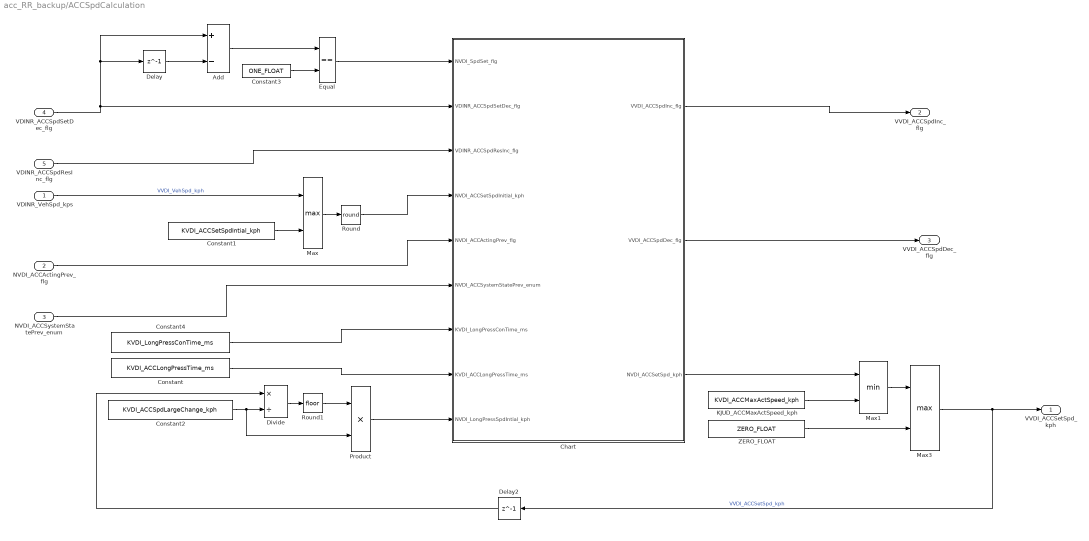
== system acc_RR_backup/ACCSpdCalculation ==
  VDINR_VehSpd_kps : Inport
  NVDI_ACCActingPrev_flg : Inport  Port=2
  NVDI_ACCSystemStatePrev_enum : Inport  Port=3
  VDINR_ACCSpdSetDec_flg : Inport  Port=4
  VDINR_ACCSpdResInc_flg : Inport  Port=5
  Add : Sum  Inputs=+-
  Chart : Stateflow chart  TreatAsAtomicUnit=on
      settings: PortSchema="{\"entries\":[{\"content\":{\"sides\":[{\"content\":{\"connectorIds\":[\"In1\",\"In2\",\"In3\",\"In4\",\"In5\",\"In6\",\"In9\",\"In7\",\"In8\"]},\"type\":\"ConnectorPlacement.EquallySpacedRectSide\",\"uuid\":\"b1b09059-7c6b-4f2a-a509-9d89abb69bff\"},{\"content\":{\"connectorIds\":[\"Out2\",\"Out3\",\"Out1\"],\"side\":\"RIGHT\"},\"type\":\"ConnectorPlacement.EquallySpacedRectSide\",\"uuid\":\"426eb2b7-8f84-437e-9ce1-b8172d5a5373\"},{\"content\":{\"connectorIds\":[],\"side\":\"TOP\"},\"type\":\"ConnectorPlacement.EquallySpacedRectSide\",\"uuid\":\"808310a0-6f78-4728-b2e8-69880cb1a9d0\"}]},\"type\":\"ConnectorPlacement.EquallySpacedConnector\",\"uuid\":\"50fcbb31-1c9a-4815-926e-b0772552613f\"}],\"packageUris\":[\"http://schema.mathworks.com/mf0/Connector/R2020b\"],\"version\":\"1.0\"}"
  Constant : Constant  Value=KVDI_ACCLongPressTime_ms
  Constant1 : Constant  Value=KVDI_ACCSetSpdIntial_kph
  Constant2 : Constant  Value=KVDI_ACCSpdLargeChange_kph
  Constant3 : Constant  Value=ONE_FLOAT
  Constant4 : Constant  Value=KVDI_LongPressConTime_ms
  Delay : Delay  DelayLength=1
  Delay2 : Delay  DelayLength=1
  Divide : Product  Inputs=*/
  Equal : RelationalOperator  Operator===  OutDataTypeStr=boolean  RndMeth=Simplest
  KJUD_ACCMaxActSpeed_kph : Constant  Value=KVDI_ACCMaxActSpeed_kph
  Max : MinMax  Function=max  Inputs=2
  Max1 : MinMax  Inputs=2
  Max3 : MinMax  Function=max  Inputs=2
  Product : Product
  Round : Rounding  Operator=round
  Round1 : Rounding
  ZERO_FLOAT : Constant  Value=ZERO_FLOAT
  VVDI_ACCSetSpd_kph : Outport
  VVDI_ACCSpdInc_flg : Outport  Port=2
  VVDI_ACCSpdDec_flg : Outport  Port=3
  wires:
  Constant4/1 -> Chart/9(KVDI_LongPressConTime_ms)
  Chart/2(VVDI_ACCSpdInc_flg) -> VVDI_ACCSpdInc_flg/1
  Chart/3(VVDI_ACCSpdDec_flg) -> VVDI_ACCSpdDec_flg/1
  Max1/1 -> Max3/1
  KJUD_ACCMaxActSpeed_kph/1 -> Max1/2
  VDINR_ACCSpdSetDec_flg/1 -> Chart/2(VDINR_ACCSpdSetDec_flg), Delay/1, Add/1
  Constant3/1 -> Equal/2
  Delay/1 -> Add/2
  Add/1 -> Equal/1
  Equal/1 -> Chart/1(NVDI_SpdSet_flg)
  ZERO_FLOAT/1 -> Max3/2
  Chart/1(NVDI_ACCSetSpd_kph) -> Max1/1
  Product/1 -> Chart/8(NVDI_LongPressSpdIntial_kph)
  Divide/1 -> Round1/1
  Round1/1 -> Product/1
  Constant2/1 -> Divide/2, Product/2
  Delay2/1 -> Divide/1
  Round/1 -> Chart/4(NVDI_ACCSetSpdInitial_kph)
  VDINR_VehSpd_kps/1 -> Max/1  "VVDI_VehSpd_kph"
  Constant1/1 -> Max/2
  Max/1 -> Round/1
  NVDI_ACCSystemStatePrev_enum/1 -> Chart/6(NVDI_ACCSystemStatePrev_enum)
  NVDI_ACCActingPrev_flg/1 -> Chart/5(NVDI_ACCActingPrev_flg)
  Max3/1 -> VVDI_ACCSetSpd_kph/1, Delay2/1  "VVDI_ACCSetSpd_kph"
  VDINR_ACCSpdResInc_flg/1 -> Chart/3(VDINR_ACCSpdResInc_flg)
  Constant/1 -> Chart/7(KVDI_ACCLongPressTime_ms)

== system acc_RR_backup/ACC_Mode_Selector ==
  ACCSetSpeed_mps : Inport
  VACCTargetVehNotAssigned_flg : Inport  Port=2
  RR : Inport  Port=3
  Vx_HV_mps : Inport  Port=4
  RV : Inport  Port=5
  Add : Sum
  Add13 : Sum  Inputs=+-
  Constant36 : Constant  Value=-0.5
  Logical Operator : Logic  Operator=OR  Inputs=3  AllPortsSameDT=off  OutDataTypeStr=boolean
  Logical Operator3 : Logic  AllPortsSameDT=off  OutDataTypeStr=boolean
  Relational Operator : RelationalOperator  Operator=<  OutDataTypeStr=boolean  RndMeth=Simplest
  Relational Operator1 : RelationalOperator  Operator=<  OutDataTypeStr=boolean  RndMeth=Simplest
  Relational Operator4 : RelationalOperator  Operator=<  OutDataTypeStr=boolean  RndMeth=Simplest
  TH_ref : Gain  Gain=1.5
  TH_ref4 : Gain  Gain=1.5
  dist_safe1 : Bias  Bias=-2
  Out1 : Outport
  wires:
  Logical Operator/1 -> Out1/1
  [Vx_PV_mps] -> Relational Operator/2
  VACCTargetVehNotAssigned_flg/1 -> Logical Operator/1
  Relational Operator/1 -> Logical Operator/2  "set_spd_compare"
  ACCSetSpeed_mps/1 -> [ACCSetSpeed_mps], Relational Operator/1
  Add/1 -> [Vx_PV_mps]
  Vx_HV_mps/1 -> [Vx_HV_mps], Add/2
  RV/1 -> Add/1
  dist_safe1/1 -> Add13/2, Relational Operator4/2  "act"
  TH_ref4/1 -> Relational Operator4/1  "des"
  Relational Operator1/1 -> Logical Operator3/1
  Constant36/1 -> Relational Operator1/2
  Add13/1 -> Relational Operator1/1
  Logical Operator3/1 -> Logical Operator/3  "dist_compare"
  RR/1 -> dist_safe1/1
  TH_ref/1 -> Add13/1  "des"
  [ACCSetSpeed_mps] -> TH_ref4/1
  [Vx_HV_mps] -> TH_ref/1
  Relational Operator4/1 -> Logical Operator3/2

== system acc_RR_backup/Latch ==
  set : Inport
  reset : Inport  Port=2
  Delay : Delay  DelayLength=1
  Logical Operator3 : Logic  AllPortsSameDT=off  OutDataTypeStr=boolean
  Logical Operator4 : Logic  Operator=NOT  AllPortsSameDT=off  OutDataTypeStr=boolean
  Switch : Switch  Criteria=u2 ~= 0
  Switch1 : Switch  Criteria=u2 ~= 0
  latched : Outport
  wires:
  Delay/1 -> Switch1/3
  Logical Operator4/1 -> Logical Operator3/2, Switch1/1
  Logical Operator3/1 -> Switch/2
  reset/1 -> Logical Operator4/1, Switch1/2
  Switch/1 -> Delay/1, latched/1
  set/1 -> Switch/1, Logical Operator3/1
  Switch1/1 -> Switch/3

== system acc_RR_backup/Smooth Switch ==
  Spd_acc_cmd : Inport
  Mode : Inport  Port=2
  TH_acc_cmd : Inport  Port=3
  TTC : Inport  Port=4
  Add12 : Sum
  Add9 : Sum  Inputs=+-
  Constant49 : Constant
  Data Type Conversion : DataTypeConversion  OutDataTypeStr=double
  Delay : Delay  DelayLength=1  InitialConditionSource=Input port  SampleTime=0.1
      settings: InputPortMap=u0,p4
  MATLAB Function : MATLAB Function  TreatAsAtomicUnit=on
  Product1 : Product
  Product2 : Product
  Scope : Scope
  Subsystem : Subsystem
  ax_cmd : Outport
  wires:
  Product2/1 -> Add12/1
  Spd_acc_cmd/1 -> Product2/1
  MATLAB Function/1(y) -> Delay/1, Scope/1, Add9/2, Product2/2
  Data Type Conversion/1 -> Delay/2, MATLAB Function/2(u)
  Constant49/1 -> Add9/1
  Product1/1 -> Add12/2
  TH_acc_cmd/1 -> Product1/2
  Add9/1 -> Product1/1
  Add12/1 -> ax_cmd/1
  Mode/1 -> Subsystem/2(Mode), Data Type Conversion/1
  Delay/1 -> MATLAB Function/3(old_u)
  Subsystem/1(Out1) -> MATLAB Function/1(tau)  "tau_selector"
  TTC/1 -> Subsystem/1(TTC)

== system acc_RR_backup/Smooth Switch1 ==
  Dynamic_cmd : Inport
  Mode : Inport  Port=2
  Kinematic_cmd : Inport  Port=3
  Add12 : Sum
  Add9 : Sum  Inputs=+-
  Constant49 : Constant
  Data Type Conversion : DataTypeConversion  OutDataTypeStr=double
  Product1 : Product
  Product2 : Product
  Transfer Fcn5 : TransferFcn  Denominator=[0.5 1]
  ax_cmd : Outport
  wires:
  Mode/1 -> Data Type Conversion/1
  Add12/1 -> ax_cmd/1
  Add9/1 -> Product1/1
  Kinematic_cmd/1 -> Product1/2
  Product1/1 -> Add12/2
  Constant49/1 -> Add9/1
  Data Type Conversion/1 -> Transfer Fcn5/1
  Transfer Fcn5/1 -> Product2/2, Add9/2
  Dynamic_cmd/1 -> Product2/1
  Product2/1 -> Add12/1
